simulink model "ysw7_2"  (R2014a)
settings: Solver=ode45  StartTime=0.0  StopTime=10.0  RelTol=1e-3
libraries: powerlib x7, dspxfrm3 x2
settings Model: Creator=Administrator  LastModifiedBy=Administrator

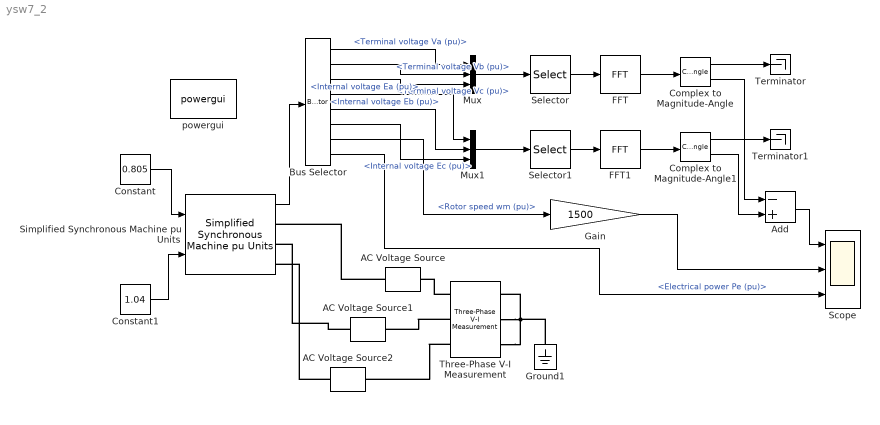
== system ysw7_2 ==
  AC Voltage Source : powerlib/Electrical Sources/AC Voltage Source  Amplitude=100  Phase=0  Frequency=50  SampleTime=0  Measurements=None
  AC Voltage Source1 : powerlib/Electrical Sources/AC Voltage Source  Amplitude=100  Phase=0  Frequency=50  SampleTime=0  Measurements=None
  AC Voltage Source2 : powerlib/Electrical Sources/AC Voltage Source  Amplitude=100  Phase=0  Frequency=50  SampleTime=0  Measurements=None
  Add : Sum  Inputs=-+
  Bus Selector : BusSelector  OutputSignals=Terminal voltage Va (pu),Terminal voltage Vb (pu),Terminal voltage Vc (pu),Internal voltage Ea (pu),Internal voltage Eb (pu),Internal voltage Ec (pu),Rotor speed wm (pu),Electrical power Pe (pu)
  Complex to Magnitude-Angle : ComplexToMagnitudeAngle
  Complex to Magnitude-Angle1 : ComplexToMagnitudeAngle
  Constant : Constant  Value=0.805
  Constant1 : Constant  Value=1.04
  FFT : dspxfrm3/FFT  CompMethod=Table lookup  TableOpt=NEW  TableOptActive=Speed  BitRevOrder=off  InheritFFTLength=on  FFTLength=64  WrapInput=on  RowConvenienceOn=on  FFTImplementation=Auto  SkipNorm=off  firstCoeffDataTypeStr=Inherit: Same word length as input  firstCoeffLastDataTypeStr=Inherit: Same word length as input  outputMin=[]  outputMax=[]  roundingMode=Floor  overflowMode=off
  FFT1 : dspxfrm3/FFT  CompMethod=Table lookup  TableOpt=NEW  TableOptActive=Speed  BitRevOrder=off  InheritFFTLength=on  FFTLength=64  WrapInput=on  RowConvenienceOn=on  FFTImplementation=Auto  SkipNorm=off  firstCoeffDataTypeStr=Inherit: Same word length as input  firstCoeffLastDataTypeStr=Inherit: Same word length as input  outputMin=[]  outputMax=[]  roundingMode=Floor  overflowMode=off
  Gain : Gain  Gain=1500
  Ground1 : powerlib/Elements/Ground  LConnTagsString=a
  Mux : Mux  Inputs=3
  Mux1 : Mux  Inputs=3
  Scope : Scope  NumInputPorts=3
      settings: YMin=-5~-5~-5  YMax=5~5~5
  Selector : Selector  InputPortWidth=3  Indices=[1]
  Selector1 : Selector  InputPortWidth=3  Indices=[1]
  Simplified Synchronous Machine pu Units : powerlib/Machines/Simplified Synchronous Machine pu Units  ConnectionType=3-wire Y  MechanicalLoad=Mechanical power Pm  MeasurementBus=off  NominalParameters=[50e6 10.5e3 50]  Mechanical=[3 28 2]  InternalRL="[0.005  0.9]"  InitialConditions="[ 0,0   0,0,0   0,0,0 ]"  Units=0  LoadFlowParameters=[1,0,0,0,0]  TsPowergui=0  TsBlock=-1  BusType=PV  Pref=0  Qref=0  Qmin=-inf  Qmax=+inf  PLF=0  QLF=0
  Terminator : Terminator
  Terminator1 : Terminator
  Three-Phase V-I Measurement : powerlib/Measurements/Three-Phase V-I Measurement  VoltageMeasurement=phase-to-ground  SetLabelV=on  LabelV=Vabc  Vpu=on  VpuLL=off  CurrentMeasurement=yes  SetLabelI=on  LabelI=Iabc  Ipu=on  Pbase=100e6  Vbase=500e3  OutputType=Complex  PhasorSimulation=off  PSBequivalent=0
  powergui : powerlib/powergui  Priority=1  SimulationMode=Continuous  SolverType=Tustin  SampleTime=50e-6  frequency=60  SPID=off  DisableSnubberDevices=off  DisableRonSwitches=off  DisableVfSwitches=off  SwTol=0  Interpol=off  DisplayEquations=off  Ts=0  methode=off  frequencyindice=50  Pbase=100e6  ErrMax=1e-4  Iterations=50  UnitsV=kV  UnitsW=MW  FunctionMessages=off  echomessages=off  HookPort=off  EnableUseOfTLC=off  x0status=blocks  RestoreLinks=warning  ResistiveCurrentMeasurement=off  Frange=[0:2:500]  Ylog=off  Xlog=on  ShowGrid=off  save=off  variable=ZData  structure=0  ZoomFFT=off  StartTime=0.0  cycles=1  DisplayStyle=1  fundamental=60  FreqAxis=off  MaxFrequency=1000  frequencyindicesteady=1  RmsSteady=1  display=off
  wires:
  Constant/1 -> Simplified Synchronous Machine pu Units/1
  Constant1/1 -> Simplified Synchronous Machine pu Units/2
  Simplified Synchronous Machine pu Units/1 -> Bus Selector/1
  Gain/1 -> Scope/2
  Selector/1 -> FFT/1
  Selector1/1 -> FFT1/1
  Add/1 -> Scope/1
  Bus Selector/7 -> Gain/1  "<Rotor speed wm (pu)>"
  Bus Selector/8 -> Scope/3  "<Electrical power Pe (pu)>"
  Mux/1 -> Selector/1
  Bus Selector/1 -> Mux/1  "<Terminal voltage Va (pu)>"
  Bus Selector/2 -> Mux/2  "<Terminal voltage Vb (pu)>"
  Bus Selector/3 -> Mux/3  "<Terminal voltage Vc (pu)>"
  Bus Selector/6 -> Mux1/3  "<Internal voltage Ec (pu)>"
  Bus Selector/5 -> Mux1/2  "<Internal voltage Eb (pu)>"
  Bus Selector/4 -> Mux1/1  "<Internal voltage Ea (pu)>"
  Mux1/1 -> Selector1/1
  FFT/1 -> Complex to Magnitude-Angle/1
  FFT1/1 -> Complex to Magnitude-Angle1/1
  Complex to Magnitude-Angle/1 -> Terminator/1
  Complex to Magnitude-Angle1/1 -> Terminator1/1
  Complex to Magnitude-Angle/2 -> Add/1
  Complex to Magnitude-Angle1/2 -> Add/2
  connections:
  AC Voltage Source/RConn1 -- Simplified Synchronous Machine pu Units/RConn1
  AC Voltage Source1/RConn1 -- Simplified Synchronous Machine pu Units/RConn2
  AC Voltage Source2/RConn1 -- Simplified Synchronous Machine pu Units/RConn3
  Three-Phase V-I Measurement/LConn1 -- AC Voltage Source/LConn1
  Three-Phase V-I Measurement/LConn2 -- AC Voltage Source1/LConn1
  Three-Phase V-I Measurement/LConn3 -- AC Voltage Source2/LConn1
  Ground1/LConn1 -- Three-Phase V-I Measurement/RConn1 -- Three-Phase V-I Measurement/RConn3 -- Three-Phase V-I Measurement/RConn2
